simulink model "bergmanGA"  (R2021a)
settings: Solver=FixedStepAuto  StartTime=0.0  StopTime=600  FixedStep=1e-2  RelTol=1e-3
values from neighbouring files (symbols this model uses):
  Gb = 153    [afterGA.m]    (also in bergmanGA.m = glucose(1); cv3.m = glucose(1); cv3a.m = glucose(1); cv4_bergman.m)
  I = ar(:,2) / 6    [cv4.m]    (also in cv4GA.m; cv4_bergman.m; cv4_bergmanGA.m; surove.m = s1.I(4001:end))
  I2 = ar2(:,2)    [cv4.m]    (also in cv4GA.m; cv4_bergman.m = ar2(:,2) / 64.4; cv4_bergmanGA.m = ar2(:,2) / 64.4)
  Ib = 12.3165    [afterGA.m]    (also in bergmanGA.m = insuline(1); cv3.m = insuline(1); cv3a.m = insuline(1); cv4.m)
  kI = 0.1645    [afterGA.m]    (also in cv4.m = Best(2); cv4GA.m = Best(2); cv4_bergman.m; cv4_bergmanGA.m)
  p2 = 0.0106    [afterGA.m]    (also in cv3.m = 0.032736; cv3a.m = 0.063098; cv4_bergman.m = Best(2) / 10; cv4_bergmanGA.m = Best(2) / 1000)
  S1b = 1.2528e4    (= 12528)    [afterGA.m]    (also in cv4.m; cv4GA.m; cv4_bergman.m; cv4_bergmanGA.m)
  S2b = S1b    (= 12528)    [afterGA.m]    (also in cv4.m; cv4GA.m; cv4_bergman.m; cv4_bergmanGA.m)
  Sg = 0.032    [afterGA.m]    (also in cv3.m = 0.030031; cv3a.m = 3.3574e-10; cv4_bergman.m = 0; cv4_bergmanGA.m = 0)
  Si = 0.00159    [afterGA.m]    (also in cv3.m = 1.0278e-13; cv3a.m = 0.00089844; cv4_bergman.m = Best(1) / 10; cv4_bergmanGA.m = Best(1) / 1000)
  T = readtable('Dat_IVGTT_RI.csv')    [bergmanGA.m]    (also in cv3.m = readtable('Dat_IVGTT_SN.csv'); cv3a.m; cv4.m = ar(:,1); cv4GA.m = ar(:,1))
  T2 = ar2(:,1)    [cv4.m]    (also in cv4GA.m; cv4_bergman.m; cv4_bergmanGA.m)
  TI = 44.55    [afterGA.m]    (also in cv4.m = Best(1); cv4GA.m = Best(1); cv4_bergman.m; cv4_bergmanGA.m)
  Vg = 1.467    [afterGA.m]    (also in cv4_bergman.m; cv4_bergmanGA.m; identik.m; lakaka.m)
  VI = 138.8    [afterGA.m]    (also in cv4.m = Best(3); cv4GA.m = Best(3); cv4_bergman.m; cv4_bergmanGA.m)
settings Model: Creator=marko  LastModifiedBy=marko

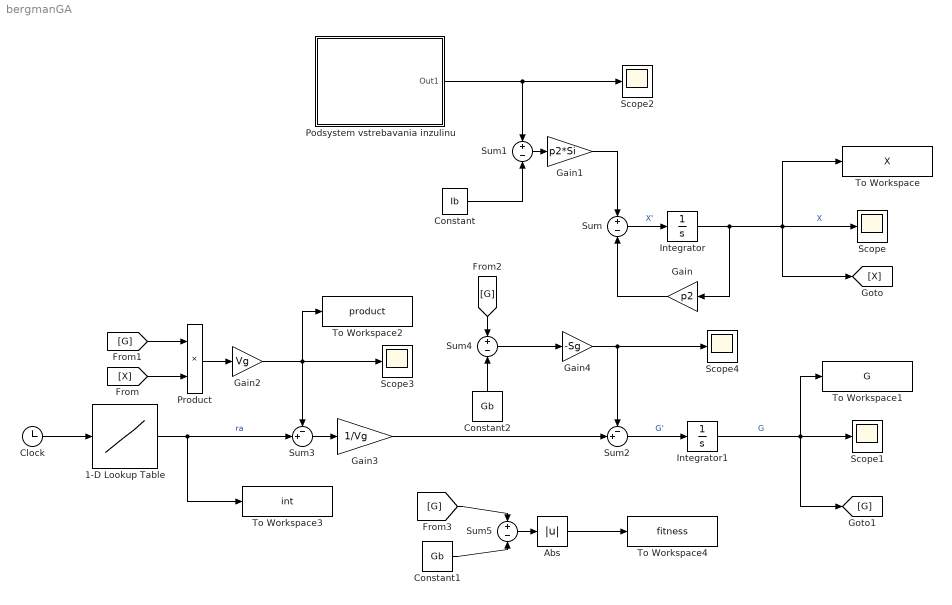
== system bergmanGA ==
  1-D Lookup Table : Lookup_n-D  NumberOfTableDimensions=1  BreakpointsForDimension1=T2  Table=I2  InternalRulePriority=Speed  RndMeth=Simplest  InputSameDT=on
  Abs : Abs
  Clock : Clock
  Constant : Constant  Value=Ib
  Constant1 : Constant  Value=Gb
  Constant2 : Constant  Value=Gb
  Gain : Gain  Gain=p2
  Gain1 : Gain  Gain=p2*Si
  Gain2 : Gain  Gain=Vg
  Gain3 : Gain  Gain=1/Vg
  Gain4 : Gain  Gain=-Sg
  Integrator : Integrator
  Integrator1 : Integrator  InitialCondition=Gb
  Podsystem vstrebavania inzulinu : Subsystem
  Product : Product
  Scope{,1..4} (5 alike) : Scope
  Sum{,1,4..5} (4 alike) : Sum  Inputs=+|-
  Sum2 : Sum  Inputs=-+|
  Sum3 : Sum  Inputs=-+|
  To Workspace : ToWorkspace  VariableName=X  SaveFormat=Timeseries  SampleTime=-1
  To Workspace1 : ToWorkspace  VariableName=G  SaveFormat=Timeseries  SampleTime=-1
  To Workspace2 : ToWorkspace  VariableName=product  SaveFormat=Timeseries  SampleTime=-1
  To Workspace3 : ToWorkspace  VariableName=int  SaveFormat=Timeseries  SampleTime=-1
  To Workspace4 : ToWorkspace  VariableName=fitness  SampleTime=-1
  wires:
  Integrator/1 -> To Workspace/1, [X], Scope/1, Gain/1  "X"
  Gain/1 -> Sum/2
  Sum/1 -> Integrator/1  "X'"
  Constant/1 -> Sum1/2
  Sum1/1 -> Gain1/1
  Gain1/1 -> Sum/1
  Integrator1/1 -> Scope1/1, [G], To Workspace1/1  "G"
  Sum2/1 -> Integrator1/1  "G'"
  Podsystem vstrebavania inzulinu/1(Out1) -> Sum1/1, Scope2/1
  Clock/1 -> 1-D Lookup Table/1
  1-D Lookup Table/1 -> To Workspace3/1, Sum3/2  "ra"
  Sum3/1 -> Gain3/1
  [G] -> Product/1
  [X] -> Product/2
  Product/1 -> Gain2/1
  Gain2/1 -> Scope3/1, To Workspace2/1, Sum3/1
  Gain3/1 -> Sum2/2
  [G] -> Sum4/1
  Constant2/1 -> Sum4/2
  Sum4/1 -> Gain4/1
  Gain4/1 -> Scope4/1, Sum2/1
  [G] -> Sum5/1
  Constant1/1 -> Sum5/2
  Sum5/1 -> Abs/1
  Abs/1 -> To Workspace4/1

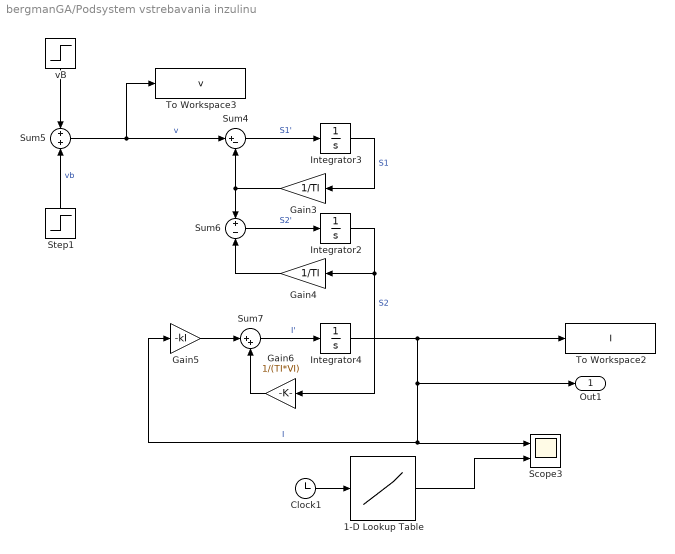
== system bergmanGA/Podsystem vstrebavania inzulinu ==
  1-D Lookup Table : Lookup_n-D  NumberOfTableDimensions=1  BreakpointsForDimension1=T  Table=I  InternalRulePriority=Speed  RndMeth=Simplest  InputSameDT=on
  Clock1 : Clock
  Gain3 : Gain  Gain=1/TI
  Gain4 : Gain  Gain=1/TI
  Gain5 : Gain  Gain=-kI
  Gain6 : Gain  Gain=1/(TI*VI)
  Integrator2 : Integrator  InitialCondition=S2b
  Integrator3 : Integrator  InitialCondition=S1b
  Integrator4 : Integrator  InitialCondition=Ib
  Scope3 : Scope  NumInputPorts=2
  Step1 : Step  Time=0  After=281.218  SampleTime=0
  Sum4 : Sum  Inputs=|+-
  Sum5 : Sum  Inputs=+|+
  Sum6 : Sum  Inputs=+|-
  Sum7 : Sum  Inputs=|++
  To Workspace2 : ToWorkspace  VariableName=I  SaveFormat=Timeseries  SampleTime=-1
  To Workspace3 : ToWorkspace  VariableName=v  SaveFormat=Timeseries  SampleTime=-1
  vB : Step  Time=5  Before=40000  After=0  SampleTime=0
  Out1 : Outport  VectorParamsAs1DForOutWhenUnconnected=off
  wires:
  Integrator4/1 -> Out1/1, Gain5/1, Scope3/1, To Workspace2/1  "I"
  vB/1 -> Sum5/1
  Gain3/1 -> Sum4/2, Sum6/1
  Gain4/1 -> Sum6/2
  1-D Lookup Table/1 -> Scope3/2
  Sum4/1 -> Integrator3/1  "S1'"
  Clock1/1 -> 1-D Lookup Table/1
  Gain5/1 -> Sum7/1
  Sum7/1 -> Integrator4/1  "I'"
  Integrator2/1 -> Gain6/1, Gain4/1  "S2"
  Sum6/1 -> Integrator2/1  "S2'"
  Gain6/1 -> Sum7/2
  Step1/1 -> Sum5/2  "vb"
  Sum5/1 -> To Workspace3/1, Sum4/1  "v"
  Integrator3/1 -> Gain3/1  "S1"
